simulink model "test"  (R2019b)
settings: Solver=VariableStepAuto  StartTime=0.0  StopTime=20.0  RelTol=1e-3
settings Model: Creator=francescoceresetti  LastModifiedBy=francescoceresetti

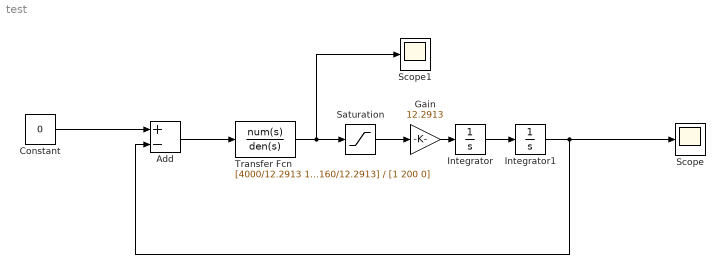
== system test ==
  Add : Sum  Inputs=+-
  Constant : Constant  Value=0
  Gain : Gain  Gain=12.2913
  Integrator : Integrator
  Integrator1 : Integrator  InitialCondition=pi/4
  Saturation : Saturate  UpperLimit=10  LowerLimit=-10
  Scope : Scope
  Scope1 : Scope
  Transfer Fcn : TransferFcn  Numerator=[4000/12.2913 1600/12.2913 160/12.2913]  Denominator=[1 200 0]
  wires:
  Integrator/1 -> Integrator1/1
  Integrator1/1 -> Add/2, Scope/1
  Transfer Fcn/1 -> Scope1/1, Saturation/1
  Saturation/1 -> Gain/1
  Gain/1 -> Integrator/1
  Add/1 -> Transfer Fcn/1
  Constant/1 -> Add/1
